simulink model "Vending_machine_implemetation2"  (R2020b)
settings: Solver=VariableStepAuto  StartTime=0.0  StopTime=10.0  RelTol=1e-3
settings Model: Creator=ADMIN  LastModifiedBy=ADMIN

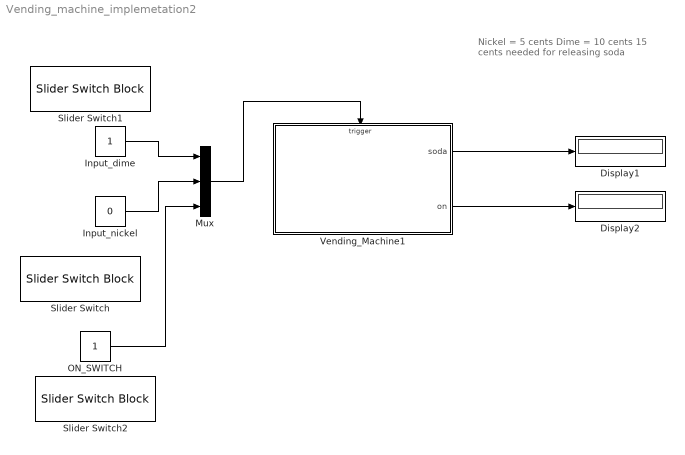
== system Vending_machine_implemetation2 ==
  note: Nickel = 5 cents
      | Dime = 10 cents
      | 15 cents needed for releasing soda
  Display1 : Display
  Display2 : Display
  Input_dime : Constant
  Input_nickel : Constant  Value=0
  Mux : Mux  Inputs=3
  ON_SWITCH : Constant
  Slider Switch : SliderSwitchBlock
      settings: Values={{'Off', 'On'}, [0 1]}
  Slider Switch1 : SliderSwitchBlock
      settings: Values={{'Off', 'On'}, [0 1]}
  Slider Switch2 : SliderSwitchBlock
      settings: Values={{'Off', 'On'}, [0 1]}
  Vending_Machine1 : Stateflow chart  TreatAsAtomicUnit=on
  wires:
  Input_nickel/1 -> Mux/2
  Vending_Machine1/2(on) -> Display2/1
  Input_dime/1 -> Mux/1
  Vending_Machine1/1(soda) -> Display1/1
  ON_SWITCH/1 -> Mux/3
  Mux/1 -> Vending_Machine1/Trigger

== stateflow chart Vending_machine_implemetation2/Vending_Machine1 ==
  settings: stateMachineType=MEALY_MACHINE
  state got_nickel
  state got_0
  state got_dime
  (default) -> got_0 : {on=1}
  got_0 -> got_nickel [order 1] : input_nickel{soda=0;}
  got_nickel -> got_0 [order 2] : input_dime{soda=1;}
  got_0 -> got_dime [order 2] : input_dime{soda=0;}
  got_dime -> got_0 [order 1] : input_nickel{soda=1;}
  got_dime -> got_nickel [order 2] : input_dime
      | {soda=1;}
  got_nickel -> got_dime [order 1] : input_nickel{soda=0;}
  data: soda output; on output
  events: input_dime input EITHER_EDGE_EVENT; input_nickel input EITHER_EDGE_EVENT; OnEvent input EITHER_EDGE_EVENT
